simulink model "simulation"  (R2015a)
settings: Solver=ode45  StartTime=0.0  StopTime=100.0  RelTol=1e-3
libraries: simulink x1
settings Model: Creator=MateusVendramini  LastModifiedBy=MateusVendramini

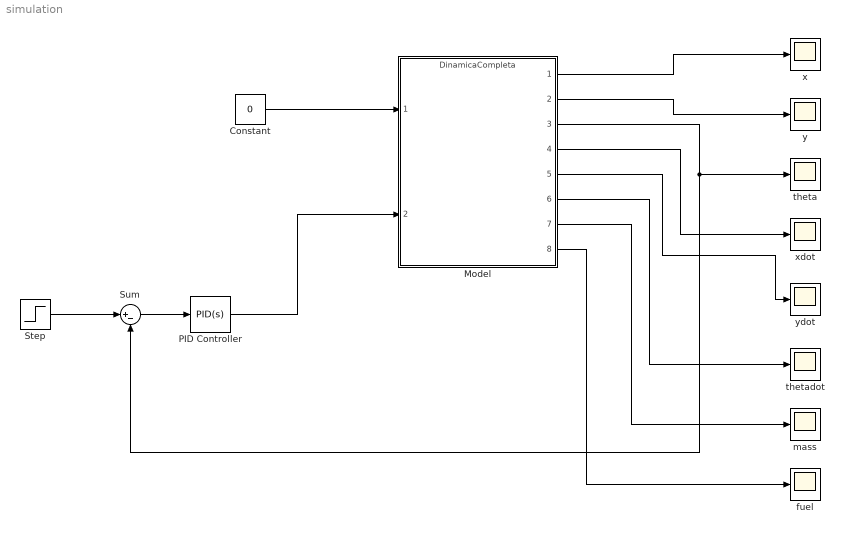
== system simulation ==
  Constant : Constant  Value=0
  Model : ModelReference  ModelNameDialog=DinamicaCompleta.slx  SimulationMode=Normal  ModelReferenceVersion=1.2  CopyOfModelName=DinamicaCompleta.slx  DefaultDataLogging=on
  PID Controller : simulink/Continuous/PID Controller  Controller=PID  TimeDomain=Continuous-time  SampleTime=-1  IntegratorMethod=Forward Euler  FilterMethod=Forward Euler  Form=Parallel  UseFilter=on  ControllerParametersSource=internal  P=5000*0.2  I=0  D=5000  N=100  InitialConditionSource=internal  InitialConditionForIntegrator=0  InitialConditionForFilter=0  ExternalReset=none  LimitOutput=off  UpperSaturationLimit=inf  LowerSaturationLimit=-inf  LinearizeAsGain=on  AntiWindupMode=none  Kb=1  TrackingMode=off  Kt=1  PParamMin=[]  PParamMax=[]  IParamMin=[]  IParamMax=[]  DParamMin=[]  DParamMax=[]  NParamMin=[]  NParamMax=[]  KbParamMin=[]  KbParamMax=[]  KtParamMin=[]  KtParamMax=[]  POutMin=[]  POutMax=[]  IOutMin=[]  IOutMax=[]  DOutMin=[]  DOutMax=[]  NOutMin=[]  NOutMax=[]  KbOutMin=[]  KbOutMax=[]  KtOutMin=[]  KtOutMax=[]  IntegratorOutMin=[]  IntegratorOutMax=[]  FilterOutMin=[]  FilterOutMax=[]  SumOutMin=[]  SumOutMax=[]  SumI1OutMin=[]  SumI1OutMax=[]  SumI2OutMin=[]  SumI2OutMax=[]  SumI3OutMin=[]  SumI3OutMax=[]  SumDOutMin=[]  SumDOutMax=[]  SaturationOutMin=[]  SaturationOutMax=[]  IntegratorContinuousStateAttributes=''  IntegratorStateMustResolveToSignalObject=off  IntegratorRTWStateStorageClass=Auto  FilterContinuousStateAttributes=''  FilterStateMustResolveToSignalObject=off  FilterRTWStateStorageClass=Auto  DifferentiatorICPrevScaledInput=0  DifferentiatorOutMin=[]  DifferentiatorOutMax=[]
  Step : Step  SampleTime=0
  Sum : Sum  Inputs=|+-
  fuel : Scope
      settings: SaveName=ScopeData7
  mass : Scope
      settings: SaveName=ScopeData6
  theta : Scope
      settings: SaveName=ScopeData2
  thetadot : Scope
      settings: SaveName=ScopeData5
  x : Scope
  xdot : Scope
      settings: SaveName=ScopeData3
  y : Scope
  ydot : Scope
      settings: SaveName=ScopeData4
  wires:
  Step/1 -> Sum/1
  Sum/1 -> PID Controller/1
  PID Controller/1 -> Model/2
  Constant/1 -> Model/1
  Model/3 -> theta/1, Sum/2
  Model/1 -> x/1
  Model/2 -> y/1
  Model/4 -> xdot/1
  Model/5 -> ydot/1
  Model/6 -> thetadot/1
  Model/7 -> mass/1
  Model/8 -> fuel/1
